simulink model "iris_opamp_layer1_16_50"  (R2023b)
settings: Solver=VariableStepAuto  StartTime=0.0  StopTime=10.0  RelTol=1e-3
libraries: vco_snn x16, dspswit3 x16, spspowerguiLib x1
settings Model: Creator=saisanjeet  LastModifiedBy=saisanjeet

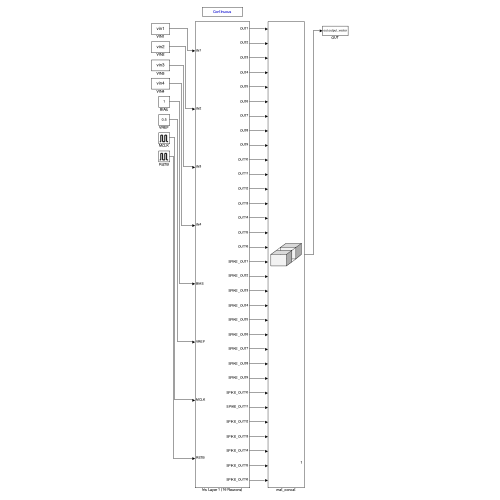
[thumbnail: Simulink's stored preview of the top-level diagram]
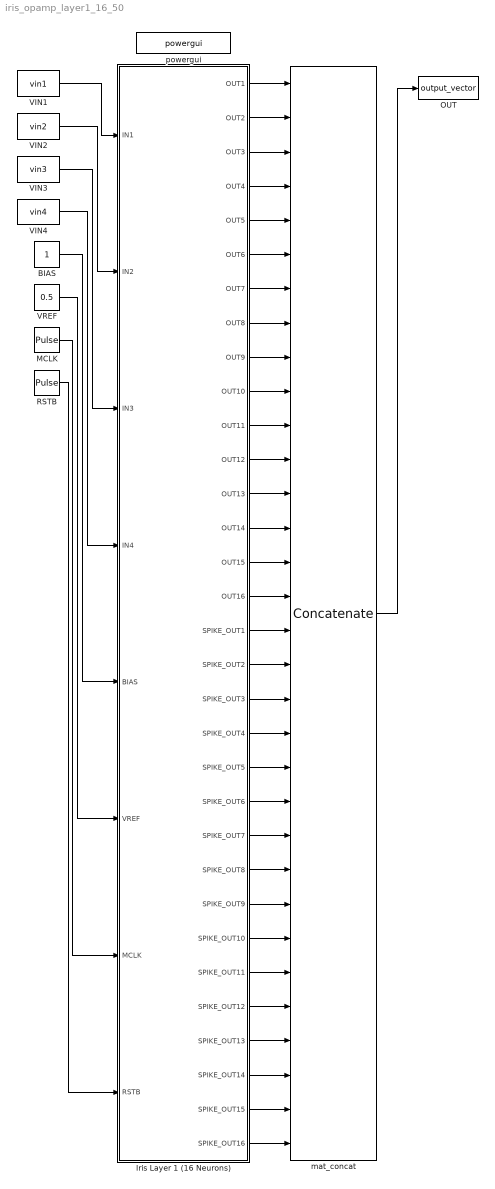
== system iris_opamp_layer1_16_50 ==
  BIAS : Constant
  Iris Layer 1 (16 Neurons) : Subsystem
  MCLK : DiscretePulseGenerator  PulseType=Time based  Period=1e-08  PulseWidth=50  PhaseDelay=1e-09
  OUT : ToWorkspace  VariableName=output_vector  SaveFormat=Timeseries  SampleTime=-1
  RSTB : DiscretePulseGenerator  PulseType=Time based  Period=4.02e-06  PulseWidth=99  PhaseDelay=1e-09
  VIN1 : FromWorkspace  VariableName=vin1  Interpolate=off  OutputAfterFinalValue=Setting to zero
  VIN2 : FromWorkspace  VariableName=vin2  Interpolate=off  OutputAfterFinalValue=Setting to zero
  VIN3 : FromWorkspace  VariableName=vin3  Interpolate=off  OutputAfterFinalValue=Setting to zero
  VIN4 : FromWorkspace  VariableName=vin4  Interpolate=off  OutputAfterFinalValue=Setting to zero
  VREF : Constant  Value=0.5
  mat_concat : Concatenate  NumInputs=32  Mode=Multidimensional array
  powergui : spspowerguiLib/powergui  Priority=1  SimulationMode=Continuous  SampleTime=50e-6  frequency=60  Iterations=50  frequencyindice=60  Pbase=100e6  ErrMax=1e-4  UnitsV=kV  UnitsW=MW  buscounter=0  FunctionMessages=off  echomessages=off  EnableUseOfTLC=off  CurrentSourceSwitches=off  DisableSnubberDevices=off  DisableRonSwitches=off  DisableVfSwitches=off  DisplayEquations=off  AutomaticDiscreteSolvers=off  SolverType=Tustin/Backward Euler (TBE)  Interpol=off  ExternalGateDelay=off  methode=off  Ts=100  x0status=blocks  SPID=on  SwTol=0  HookPort=off  NonlinearTolerance=1e-4  nMaxIteration=100  ContinueOnMaxIteration=off  RestoreLinks=warning  ResistiveCurrentMeasurement=off  Frange=[0:2:500]  Ylog=off  Xlog=on  ShowGrid=off  save=off  variable=ZData  structure=0  ZoomFFT=off  StartTime=0.0  cycles=1  DisplayStyle=1  fundamental=60  FreqAxis=off  MaxFrequency=1000  frequencyindicesteady=1  RmsSteady=1  display=off
  wires:
  VIN1/1 -> Iris Layer 1 (16 Neurons)/1(IN1)
  VIN2/1 -> Iris Layer 1 (16 Neurons)/2(IN2)
  VIN3/1 -> Iris Layer 1 (16 Neurons)/3(IN3)
  VIN4/1 -> Iris Layer 1 (16 Neurons)/4(IN4)
  BIAS/1 -> Iris Layer 1 (16 Neurons)/5(BIAS)
  VREF/1 -> Iris Layer 1 (16 Neurons)/6(VREF)
  MCLK/1 -> Iris Layer 1 (16 Neurons)/7(MCLK)
  RSTB/1 -> Iris Layer 1 (16 Neurons)/8(RSTB)
  Iris Layer 1 (16 Neurons)/1(OUT1) -> mat_concat/1
  Iris Layer 1 (16 Neurons)/17(SPIKE_OUT1) -> mat_concat/17
  Iris Layer 1 (16 Neurons)/2(OUT2) -> mat_concat/2
  Iris Layer 1 (16 Neurons)/18(SPIKE_OUT2) -> mat_concat/18
  Iris Layer 1 (16 Neurons)/3(OUT3) -> mat_concat/3
  Iris Layer 1 (16 Neurons)/19(SPIKE_OUT3) -> mat_concat/19
  Iris Layer 1 (16 Neurons)/4(OUT4) -> mat_concat/4
  Iris Layer 1 (16 Neurons)/20(SPIKE_OUT4) -> mat_concat/20
  Iris Layer 1 (16 Neurons)/5(OUT5) -> mat_concat/5
  Iris Layer 1 (16 Neurons)/21(SPIKE_OUT5) -> mat_concat/21
  Iris Layer 1 (16 Neurons)/6(OUT6) -> mat_concat/6
  Iris Layer 1 (16 Neurons)/22(SPIKE_OUT6) -> mat_concat/22
  Iris Layer 1 (16 Neurons)/7(OUT7) -> mat_concat/7
  Iris Layer 1 (16 Neurons)/23(SPIKE_OUT7) -> mat_concat/23
  Iris Layer 1 (16 Neurons)/8(OUT8) -> mat_concat/8
  Iris Layer 1 (16 Neurons)/24(SPIKE_OUT8) -> mat_concat/24
  Iris Layer 1 (16 Neurons)/9(OUT9) -> mat_concat/9
  Iris Layer 1 (16 Neurons)/25(SPIKE_OUT9) -> mat_concat/25
  Iris Layer 1 (16 Neurons)/10(OUT10) -> mat_concat/10
  Iris Layer 1 (16 Neurons)/26(SPIKE_OUT10) -> mat_concat/26
  Iris Layer 1 (16 Neurons)/11(OUT11) -> mat_concat/11
  Iris Layer 1 (16 Neurons)/27(SPIKE_OUT11) -> mat_concat/27
  Iris Layer 1 (16 Neurons)/12(OUT12) -> mat_concat/12
  Iris Layer 1 (16 Neurons)/28(SPIKE_OUT12) -> mat_concat/28
  Iris Layer 1 (16 Neurons)/13(OUT13) -> mat_concat/13
  Iris Layer 1 (16 Neurons)/29(SPIKE_OUT13) -> mat_concat/29
  Iris Layer 1 (16 Neurons)/14(OUT14) -> mat_concat/14
  Iris Layer 1 (16 Neurons)/30(SPIKE_OUT14) -> mat_concat/30
  Iris Layer 1 (16 Neurons)/15(OUT15) -> mat_concat/15
  Iris Layer 1 (16 Neurons)/31(SPIKE_OUT15) -> mat_concat/31
  Iris Layer 1 (16 Neurons)/16(OUT16) -> mat_concat/16
  Iris Layer 1 (16 Neurons)/32(SPIKE_OUT16) -> mat_concat/32
  mat_concat/1 -> OUT/1

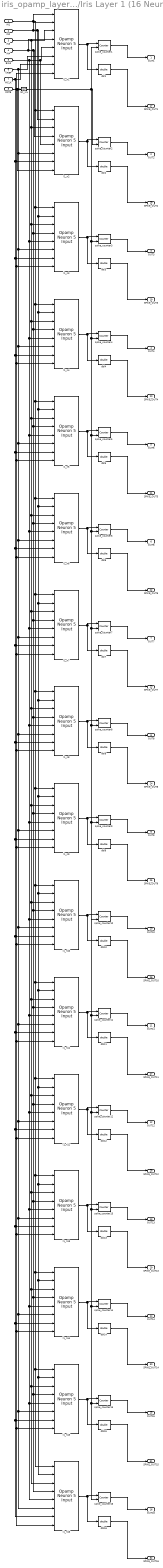
== system iris_opamp_layer1_16_50/Iris Layer 1 (16 Neurons) ==
  IN1 : Inport
  IN2 : Inport  Port=2
  IN3 : Inport  Port=3
  IN4 : Inport  Port=4
  BIAS : Inport  Port=5
  VREF : Inport  Port=6
  MCLK : Inport  Port=7
  RSTB : Inport  Port=8
  dbl{1..16} (16 alike) : DataTypeConversion  OutDataTypeStr=double  SaturateOnIntegerOverflow=off  RndMeth=Floor
  l1_n1 : vco_snn/Opamp Neuron 5 Input  rf=50000  cf=1e-12  vth=0.4  vcm=0.5  spike_amp=0.2  rin1=17174.7695  spike_sign1=1  rin2=27760.0293  spike_sign2=-1  rin3=79506.9297  spike_sign3=-1  rin4=19601.2539  spike_sign4=1  rin5=5e+19  spike_sign5=0
  l1_n10 : vco_snn/Opamp Neuron 5 Input  rf=50000  cf=1e-12  vth=0.4  vcm=0.5  spike_amp=0.2  rin1=10960.5342  spike_sign1=1  rin2=64491.4648  spike_sign2=-1  rin3=23158.7324  spike_sign3=1  rin4=22302.0996  spike_sign4=-1  rin5=5e+19  spike_sign5=0
  l1_n11 : vco_snn/Opamp Neuron 5 Input  rf=50000  cf=1e-12  vth=0.4  vcm=0.5  spike_amp=0.2  rin1=9178.626  spike_sign1=1  rin2=34174.0156  spike_sign2=-1  rin3=11737.0049  spike_sign3=1  rin4=92255.0391  spike_sign4=1  rin5=5e+19  spike_sign5=0
  l1_n12 : vco_snn/Opamp Neuron 5 Input  rf=50000  cf=1e-12  vth=0.4  vcm=0.5  spike_amp=0.2  rin1=20246.9219  spike_sign1=-1  rin2=20311.3203  spike_sign2=1  rin3=21970.0391  spike_sign3=-1  rin4=24619.0352  spike_sign4=1  rin5=5e+19  spike_sign5=0
  l1_n13 : vco_snn/Opamp Neuron 5 Input  rf=50000  cf=1e-12  vth=0.4  vcm=0.5  spike_amp=0.2  rin1=77740.2188  spike_sign1=-1  rin2=153128.6719  spike_sign2=1  rin3=12191.9492  spike_sign3=-1  rin4=29177.5664  spike_sign4=-1  rin5=5e+19  spike_sign5=0
  l1_n14 : vco_snn/Opamp Neuron 5 Input  rf=50000  cf=1e-12  vth=0.4  vcm=0.5  spike_amp=0.2  rin1=15672.1611  spike_sign1=1  rin2=61745.1484  spike_sign2=-1  rin3=9142.9229  spike_sign3=1  rin4=11324.6514  spike_sign4=1  rin5=5e+19  spike_sign5=0
  l1_n15 : vco_snn/Opamp Neuron 5 Input  rf=50000  cf=1e-12  vth=0.4  vcm=0.5  spike_amp=0.2  rin1=227968.4844  spike_sign1=1  rin2=18015.1406  spike_sign2=-1  rin3=14847.2578  spike_sign3=1  rin4=29353.8457  spike_sign4=1  rin5=5e+19  spike_sign5=0
  l1_n16 : vco_snn/Opamp Neuron 5 Input  rf=50000  cf=1e-12  vth=0.4  vcm=0.5  spike_amp=0.2  rin1=17155.4531  spike_sign1=-1  rin2=14833.9775  spike_sign2=1  rin3=14818.6631  spike_sign3=1  rin4=10387.9648  spike_sign4=1  rin5=5e+19  spike_sign5=0
  l1_n2 : vco_snn/Opamp Neuron 5 Input  rf=50000  cf=1e-12  vth=0.4  vcm=0.5  spike_amp=0.2  rin1=11493.1836  spike_sign1=-1  rin2=15764.4072  spike_sign2=1  rin3=89218.6172  spike_sign3=-1  rin4=15840.665  spike_sign4=1  rin5=5e+19  spike_sign5=0
  l1_n3 : vco_snn/Opamp Neuron 5 Input  rf=50000  cf=1e-12  vth=0.4  vcm=0.5  spike_amp=0.2  rin1=43367.3477  spike_sign1=1  rin2=678119.75  spike_sign2=-1  rin3=29469.6348  spike_sign3=1  rin4=109223.0156  spike_sign4=1  rin5=5e+19  spike_sign5=0
  l1_n4 : vco_snn/Opamp Neuron 5 Input  rf=50000  cf=1e-12  vth=0.4  vcm=0.5  spike_amp=0.2  rin1=23059.168  spike_sign1=1  rin2=30238.3848  spike_sign2=-1  rin3=1037485.3125  spike_sign3=1  rin4=2163092.25  spike_sign4=-1  rin5=5e+19  spike_sign5=0
  l1_n5 : vco_snn/Opamp Neuron 5 Input  rf=50000  cf=1e-12  vth=0.4  vcm=0.5  spike_amp=0.2  rin1=45610.0625  spike_sign1=1  rin2=116946.6016  spike_sign2=1  rin3=10947.3564  spike_sign3=1  rin4=30880.0176  spike_sign4=1  rin5=5e+19  spike_sign5=0
  l1_n6 : vco_snn/Opamp Neuron 5 Input  rf=50000  cf=1e-12  vth=0.4  vcm=0.5  spike_amp=0.2  rin1=42143.0547  spike_sign1=-1  rin2=21689.166  spike_sign2=-1  rin3=205254.5156  spike_sign3=-1  rin4=31082.9492  spike_sign4=-1  rin5=5e+19  spike_sign5=0
  l1_n7 : vco_snn/Opamp Neuron 5 Input  rf=50000  cf=1e-12  vth=0.4  vcm=0.5  spike_amp=0.2  rin1=35843.707  spike_sign1=-1  rin2=166711.8125  spike_sign2=1  rin3=15399.2832  spike_sign3=1  rin4=16220.2354  spike_sign4=1  rin5=5e+19  spike_sign5=0
  l1_n8 : vco_snn/Opamp Neuron 5 Input  rf=50000  cf=1e-12  vth=0.4  vcm=0.5  spike_amp=0.2  rin1=11209.7188  spike_sign1=-1  rin2=13870.9795  spike_sign2=1  rin3=29750.1855  spike_sign3=1  rin4=10357.917  spike_sign4=1  rin5=5e+19  spike_sign5=0
  l1_n9 : vco_snn/Opamp Neuron 5 Input  rf=50000  cf=1e-12  vth=0.4  vcm=0.5  spike_amp=0.2  rin1=14498.9883  spike_sign1=1  rin2=10993.2852  spike_sign2=-1  rin3=11117.5508  spike_sign3=-1  rin4=24906.3887  spike_sign4=-1  rin5=5e+19  spike_sign5=0
  rst_inv : Logic  Operator=NOT  IconShape=distinctive  AllPortsSameDT=off  OutDataTypeStr=boolean
  spike_counter{1..16} (16 alike) : dspswit3/Counter  Direction=Up  CountEvent=Rising edge  CounterSize=User defined  MaxCount=1024  InitialCount=0  Output=Count  HitValue=32  ResetInput=on  SamplesPerFrame=1  Ts=1  CntDtype=double  HitDtype=Logical
  OUT1 : Outport
  OUT2 : Outport  Port=2
  OUT3 : Outport  Port=3
  OUT4 : Outport  Port=4
  OUT5 : Outport  Port=5
  OUT6 : Outport  Port=6
  OUT7 : Outport  Port=7
  OUT8 : Outport  Port=8
  OUT9 : Outport  Port=9
  OUT10 : Outport  Port=10
  OUT11 : Outport  Port=11
  OUT12 : Outport  Port=12
  OUT13 : Outport  Port=13
  OUT14 : Outport  Port=14
  OUT15 : Outport  Port=15
  OUT16 : Outport  Port=16
  SPIKE_OUT1 : Outport  Port=17
  SPIKE_OUT2 : Outport  Port=18
  SPIKE_OUT3 : Outport  Port=19
  SPIKE_OUT4 : Outport  Port=20
  SPIKE_OUT5 : Outport  Port=21
  SPIKE_OUT6 : Outport  Port=22
  SPIKE_OUT7 : Outport  Port=23
  SPIKE_OUT8 : Outport  Port=24
  SPIKE_OUT9 : Outport  Port=25
  SPIKE_OUT10 : Outport  Port=26
  SPIKE_OUT11 : Outport  Port=27
  SPIKE_OUT12 : Outport  Port=28
  SPIKE_OUT13 : Outport  Port=29
  SPIKE_OUT14 : Outport  Port=30
  SPIKE_OUT15 : Outport  Port=31
  SPIKE_OUT16 : Outport  Port=32
  wires:
  spike_counter11/1 -> OUT11/1
  dbl14/1 -> SPIKE_OUT14/1
  spike_counter3/1 -> OUT3/1
  spike_counter13/1 -> OUT13/1
  dbl12/1 -> SPIKE_OUT12/1
  spike_counter5/1 -> OUT5/1
  dbl6/1 -> SPIKE_OUT6/1
  spike_counter4/1 -> OUT4/1
  spike_counter7/1 -> OUT7/1
  dbl5/1 -> SPIKE_OUT5/1
  spike_counter15/1 -> OUT15/1
  VREF/1 -> l1_n15/6, l1_n16/6, l1_n14/6, l1_n13/6, l1_n12/6, l1_n11/6, l1_n10/6, l1_n9/6, l1_n8/6, l1_n7/6, l1_n6/6, l1_n5/6, l1_n4/6, l1_n3/6, l1_n2/6, l1_n1/6
  l1_n14/1 -> spike_counter14/1, dbl14/1
  dbl15/1 -> SPIKE_OUT15/1
  IN1/1 -> l1_n15/1, l1_n16/1, l1_n14/1, l1_n13/1, l1_n12/1, l1_n11/1, l1_n10/1, l1_n9/1, l1_n8/1, l1_n7/1, l1_n6/1, l1_n5/1, l1_n4/1, l1_n3/1, l1_n2/1, l1_n1/1
  dbl4/1 -> SPIKE_OUT4/1
  l1_n7/1 -> spike_counter7/1, dbl7/1
  l1_n3/1 -> spike_counter3/1, dbl3/1
  spike_counter6/1 -> OUT6/1
  spike_counter2/1 -> OUT2/1
  spike_counter8/1 -> OUT8/1
  l1_n10/1 -> spike_counter10/1, dbl10/1
  spike_counter10/1 -> OUT10/1
  l1_n4/1 -> spike_counter4/1, dbl4/1
  l1_n5/1 -> spike_counter5/1, dbl5/1
  spike_counter14/1 -> OUT14/1
  spike_counter1/1 -> OUT1/1
  l1_n9/1 -> spike_counter9/1, dbl9/1
  dbl8/1 -> SPIKE_OUT8/1
  dbl9/1 -> SPIKE_OUT9/1
  IN2/1 -> l1_n15/2, l1_n16/2, l1_n14/2, l1_n13/2, l1_n12/2, l1_n11/2, l1_n10/2, l1_n9/2, l1_n8/2, l1_n7/2, l1_n6/2, l1_n5/2, l1_n4/2, l1_n3/2, l1_n2/2, l1_n1/2
  l1_n12/1 -> spike_counter12/1, dbl12/1
  dbl1/1 -> SPIKE_OUT1/1
  spike_counter9/1 -> OUT9/1
  IN4/1 -> l1_n15/4, l1_n16/4, l1_n14/4, l1_n13/4, l1_n12/4, l1_n11/4, l1_n10/4, l1_n9/4, l1_n8/4, l1_n7/4, l1_n6/4, l1_n5/4, l1_n4/4, l1_n3/4, l1_n2/4, l1_n1/4
  MCLK/1 -> l1_n15/7, l1_n16/7, l1_n14/7, l1_n13/7, l1_n12/7, l1_n11/7, l1_n10/7, l1_n9/7, l1_n8/7, l1_n7/7, l1_n6/7, l1_n5/7, l1_n4/7, l1_n3/7, l1_n2/7, l1_n1/7
  BIAS/1 -> l1_n15/5, l1_n16/5, l1_n14/5, l1_n13/5, l1_n12/5, l1_n11/5, l1_n10/5, l1_n9/5, l1_n8/5, l1_n7/5, l1_n6/5, l1_n5/5, l1_n4/5, l1_n3/5, l1_n1/5, l1_n2/5
  l1_n6/1 -> spike_counter6/1, dbl6/1
  dbl16/1 -> SPIKE_OUT16/1
  l1_n1/1 -> spike_counter1/1, dbl1/1
  l1_n15/1 -> spike_counter15/1, dbl15/1
  l1_n2/1 -> spike_counter2/1, dbl2/1
  dbl7/1 -> SPIKE_OUT7/1
  dbl3/1 -> SPIKE_OUT3/1
  dbl11/1 -> SPIKE_OUT11/1
  IN3/1 -> l1_n15/3, l1_n16/3, l1_n14/3, l1_n13/3, l1_n12/3, l1_n11/3, l1_n10/3, l1_n9/3, l1_n8/3, l1_n7/3, l1_n6/3, l1_n5/3, l1_n4/3, l1_n3/3, l1_n2/3, l1_n1/3
  dbl2/1 -> SPIKE_OUT2/1
  spike_counter16/1 -> OUT16/1
  RSTB/1 -> l1_n15/8, l1_n16/8, l1_n14/8, l1_n13/8, l1_n12/8, l1_n11/8, l1_n10/8, l1_n9/8, l1_n8/8, l1_n7/8, l1_n6/8, l1_n5/8, l1_n4/8, l1_n3/8, rst_inv/1, l1_n2/8, l1_n1/8
  l1_n16/1 -> spike_counter16/1, dbl16/1
  l1_n8/1 -> spike_counter8/1, dbl8/1
  rst_inv/1 -> spike_counter15/2, spike_counter16/2, spike_counter14/2, spike_counter13/2, spike_counter12/2, spike_counter11/2, spike_counter9/2, spike_counter10/2, spike_counter8/2, spike_counter7/2, spike_counter6/2, spike_counter5/2, spike_counter4/2, spike_counter3/2, spike_counter1/2, spike_counter2/2
  dbl13/1 -> SPIKE_OUT13/1
  dbl10/1 -> SPIKE_OUT10/1
  spike_counter12/1 -> OUT12/1
  l1_n13/1 -> spike_counter13/1, dbl13/1
  l1_n11/1 -> spike_counter11/1, dbl11/1
